simulink model "TRN_V3_CodeGen"  (R2022a)
settings: Solver=FixedStepAuto  StartTime=0.0  StopTime=300  FixedStep=0.04  RelTol=1e-3
PreLoadFcn:
  | % Add DataBus Path
  | addpath(',/TRN');
  | addpath('./MAP/');
  | addpath('./MAP/MAP_DB');
  | addpath('./MAP/DVOF');
  | addpath(genpath(cd));
  | load('BusStructureTRN.mat');
InitFcn:
  | % Add DataBus Path
  | addpath(',/TRN');
  | addpath('./MAP/');
  | addpath('./MAP/MAP_DB');
  | addpath('./MAP/DVOF');
  | addpath(genpath(cd));
  | load('BusStructureTRN.mat');
undefined symbols (not defined in the file or in its folder): Altitude_INS, INSDataNotValid, Latitude_INS, Longitude_INS, RALTValid, TRN, TRNlib
libraries: simulink_extras x33, aerolibconvert2 x6, dspstat3 x3, sharedtransform x2
(part 2 of 3)

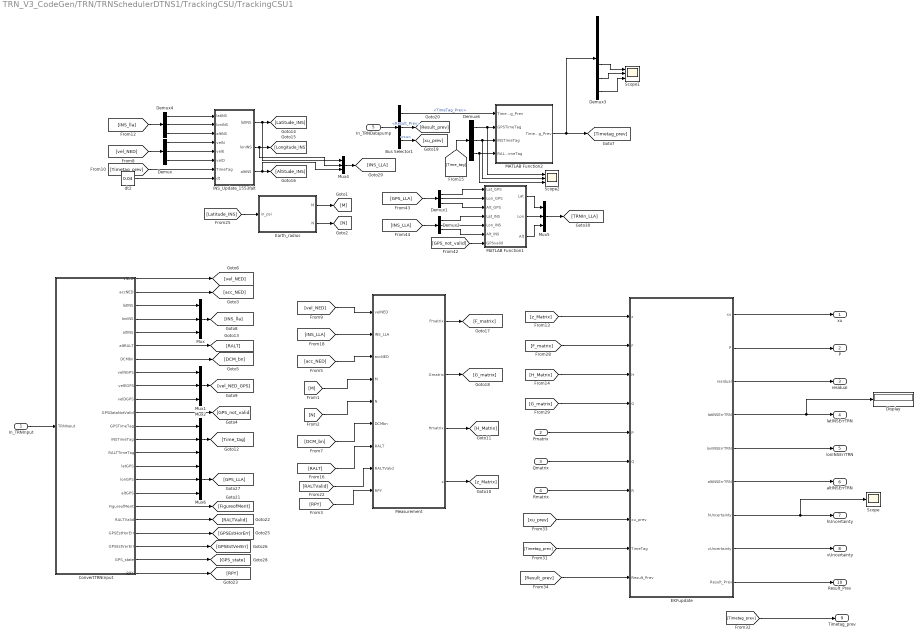
== system TRN_V3_CodeGen/TRN/TRNSchedulerDTNS1/TrackingCSU/TrackingCSU1 ==
  In_TRNInput : Inport  OutDataTypeStr=Bus: TRNInput
  Pmatrix : Inport  Port=2
  Qmatrix : Inport  Port=3
  Rmatrix : Inport  Port=4
  In_TRNDatapump : Inport  Port=5  OutDataTypeStr=Bus: TRNDatapump  PortDimensions=1
  Bus Selector1 : BusSelector  OutputSignals=TimeTag_Prev,Result_Prev,xu
  ConvertTRNInput : Subsystem  TreatAsAtomicUnit=on
  Demux{,1..2,4,6} (5 alike) : Demux  Outputs=3
  Demux3 : Demux  Outputs=6
  Display : Display
  EKFupdate : Subsystem
  Earth_radius : MATLAB Function  TreatAsAtomicUnit=on
  INS_Update_1553falt : MATLAB Function  TreatAsAtomicUnit=on
  MATLAB Function1 : MATLAB Function  TreatAsAtomicUnit=on
  MATLAB Function2 : MATLAB Function  TreatAsAtomicUnit=on
  Measurement : Subsystem
  Mux{,1..2,4..6} (6 alike) : Mux  Inputs=3
  Scope : Scope
  Scope1 : Scope  NumInputPorts=3
  Scope2 : Scope  NumInputPorts=3
  dt2 : Constant  Value=0.04  OutDataTypeStr=double
  xu : Outport
  P : Outport  Port=2
  residual : Outport  Port=3
  latINSErrTRN : Outport  Port=4
  lonINSErrTRN : Outport  Port=5
  altINSErrTRN : Outport  Port=6
  hUncertainty : Outport  Port=7
  vUncertainty : Outport  Port=8
  Timetag_prev : Outport  Port=9
  Result_Prev : Outport  Port=10
  wires:
  Mux5/1 -> [TRNIn_LLA]
  MATLAB Function1/3(Alt) -> Mux5/3
  MATLAB Function1/1(Lat) -> Mux5/1
  MATLAB Function1/2(Lon) -> Mux5/2
  Demux2/3 -> MATLAB Function1/6(Alt_INS)
  Demux2/2 -> MATLAB Function1/5(Lon_INS)
  Demux2/1 -> MATLAB Function1/4(Lat_INS)
  [INS_LLA] -> Demux2/1
  Mux4/1 -> [INS_LLA]
  Demux1/3 -> MATLAB Function1/3(Alt_GPS)
  Demux1/1 -> MATLAB Function1/1(Lat_GPS)
  Demux1/2 -> MATLAB Function1/2(Lon_GPS)
  [GPS_LLA] -> Demux1/1
  [GPS_not_valid] -> MATLAB Function1/7(GPSvalid)
  ConvertTRNInput/22(GPS_state) -> [GPS_state]
  ConvertTRNInput/21(GPSEstVerErr) -> [GPSEstVerErr]
  ConvertTRNInput/20(GPSEstHorErr) -> [GPSEstHorErr]
  Demux/3 -> INS_Update_1553falt/6(velD)
  Demux/1 -> INS_Update_1553falt/4(velN)
  Demux/2 -> INS_Update_1553falt/5(velE)
  dt2/1 -> INS_Update_1553falt/8(dt)
  Bus Selector1/1 -> MATLAB Function2/1("TimeTag_Prev ")  "<TimeTag_Prev>"
  In_TRNDatapump/1 -> Bus Selector1/1
  INS_Update_1553falt/3(altINS) -> [Altitude_INS], Mux4/3
  In_TRNInput/1 -> ConvertTRNInput/1(TRNInput)
  INS_Update_1553falt/1(latINS) -> [Latitude_INS], Mux4/1
  INS_Update_1553falt/2(lonINS) -> [Longitude_INS], Mux4/2
  ConvertTRNInput/2(accNED) -> [acc_NED]
  ConvertTRNInput/11(GPSDataNotValid) -> [GPS_not_valid]
  ConvertTRNInput/7(DCMbn) -> [DCM_bn]
  ConvertTRNInput/1(vNED) -> [vel_NED]
  [vel_NED] -> Demux/1
  [Timetag_prev] -> INS_Update_1553falt/7(TimeTag)
  ConvertTRNInput/3(latINS) -> Mux/1
  ConvertTRNInput/4(lonINS) -> Mux/2
  ConvertTRNInput/5(altINS) -> Mux/3
  Mux/1 -> [INS_lla]
  [INS_lla] -> Demux4/1
  Demux4/2 -> INS_Update_1553falt/2("lonINS ")
  Demux4/1 -> INS_Update_1553falt/1("latINS ")
  Demux4/3 -> INS_Update_1553falt/3("altINS ")
  ConvertTRNInput/10(velDGPS) -> Mux1/3
  ConvertTRNInput/9(velEGPS) -> Mux1/2
  Mux1/1 -> [vel_NED_GPS]
  ConvertTRNInput/8(velNGPS) -> Mux1/1
  Mux2/1 -> [Time_tag]
  ConvertTRNInput/12(GPSTimeTag) -> Mux2/1
  ConvertTRNInput/13(INSTimeTag) -> Mux2/2
  ConvertTRNInput/14(RALTTimeTag) -> Mux2/3
  [Time_tag] -> Demux6/1
  Demux6/1 -> Scope2/1, MATLAB Function2/2(GPSTimeTag)
  Demux6/2 -> Scope2/2, MATLAB Function2/3(INSTimeTag)
  Demux6/3 -> Scope2/3, MATLAB Function2/4(RALTTimeTag)
  ConvertTRNInput/6(altRALT) -> [RALT]
  [Timetag_prev] -> Timetag_prev/1
  Bus Selector1/3 -> [xu_prev]  "<xu>"
  Bus Selector1/2 -> [Result_prev]  "<Result_Prev>"
  Measurement/1(Fmatrix) -> [F_matrix]
  Measurement/2(Gmatrix) -> [G_matrix]
  Measurement/3(Hmatrix) -> [H_Matrix]
  Measurement/4(z) -> [z_Matrix]
  [z_Matrix] -> EKFupdate/1(z)
  [F_matrix] -> EKFupdate/2(F)
  [H_Matrix] -> EKFupdate/3(H)
  [G_matrix] -> EKFupdate/4(G)
  Pmatrix/1 -> EKFupdate/5("P ")
  Qmatrix/1 -> EKFupdate/6(Q)
  Rmatrix/1 -> EKFupdate/7(R)
  [xu_prev] -> EKFupdate/8(xu_prev)
  [Timetag_prev] -> EKFupdate/9(TimeTag)
  [Result_prev] -> EKFupdate/10("Result_Prev ")
  EKFupdate/1(xu) -> xu/1
  EKFupdate/2(P) -> P/1
  EKFupdate/3(residual) -> residual/1
  EKFupdate/8(vUncertainty) -> vUncertainty/1
  EKFupdate/4(latINSErrTRN) -> Display/1, latINSErrTRN/1
  EKFupdate/5(lonINSErrTRN) -> lonINSErrTRN/1
  EKFupdate/6(altINSErrTRN) -> altINSErrTRN/1
  EKFupdate/9(Result_Prev) -> Result_Prev/1
  ConvertTRNInput/18(FigureofMerit) -> [FigureofMerit]
  EKFupdate/7(hUncertainty) -> Scope/1, hUncertainty/1
  ConvertTRNInput/19(RALTValid) -> [RALTValid]
  [RALTValid] -> Measurement/8(RALTValid)
  [vel_NED] -> Measurement/1(velNED)
  [INS_LLA] -> Measurement/2(INS_LLA)
  [acc_NED] -> Measurement/3(accNED)
  [M] -> Measurement/4(M)
  [N] -> Measurement/5(N)
  [Latitude_INS] -> Earth_radius/1(in_psi)
  Earth_radius/1(M) -> [M]
  Earth_radius/2(N) -> [N]
  ConvertTRNInput/15(latGPS) -> Mux6/1
  ConvertTRNInput/16(lonGPS) -> Mux6/2
  ConvertTRNInput/17(altGPS) -> Mux6/3
  Mux6/1 -> [GPS_LLA]
  [RALT] -> Measurement/7(RALT)
  [DCM_bn] -> Measurement/6(DCMbn)
  ConvertTRNInput/23(RPY) -> [RPY]
  [RPY] -> Measurement/9(RPY)
  MATLAB Function2/1(TimeTag_Prev) -> Demux3/1, [Timetag_prev]
  Demux3/4 -> Scope1/1
  Demux3/5 -> Scope1/2
  Demux3/6 -> Scope1/3

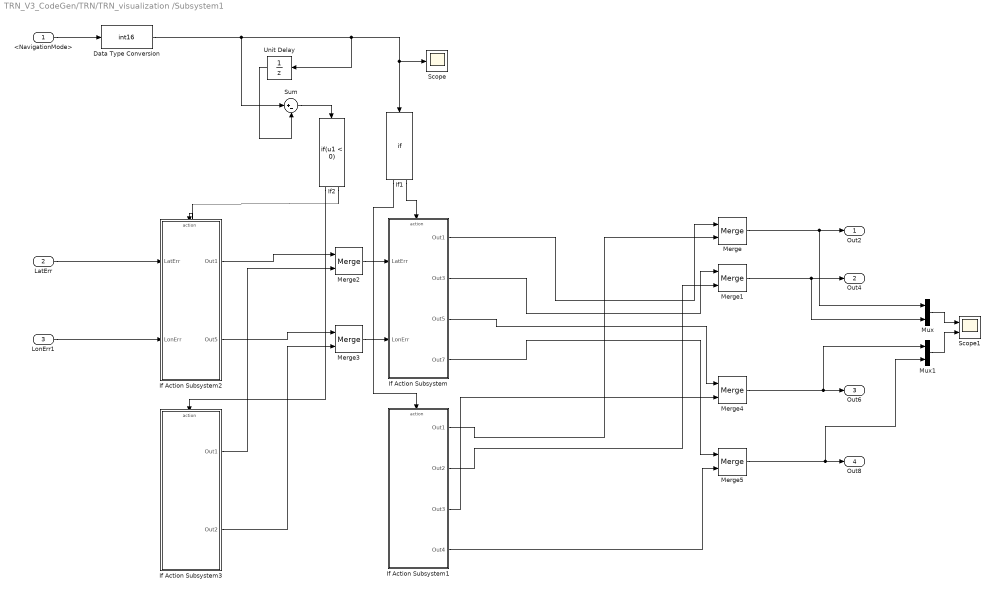
== system TRN_V3_CodeGen/TRN/TRN_visualization /Subsystem1 ==
  <NavigationMode> : Inport
  LatErr : Inport  Port=2
  LonErr1 : Inport  Port=3
  Data Type Conversion : DataTypeConversion  OutDataTypeStr=int16  SaturateOnIntegerOverflow=off  RndMeth=Floor
  If Action Subsystem : Subsystem  TreatAsAtomicUnit=on
  If Action Subsystem1 : Subsystem  TreatAsAtomicUnit=on
  If Action Subsystem2 : Subsystem  TreatAsAtomicUnit=on
  If Action Subsystem3 : Subsystem  TreatAsAtomicUnit=on
  If1 : If
  If2 : If  IfExpression=u1 < 0
  Merge{,1..5} (6 alike) : Merge
  Mux : Mux  Inputs=2
  Mux1 : Mux  Inputs=2
  Scope : Scope
  Scope1 : Scope  NumInputPorts=2
  Sum : Sum  Inputs=|+-
  Unit Delay : UnitDelay  SampleTime=-1  HasFrameUpgradeWarning=on
  Out2 : Outport
  Out4 : Outport  Port=2
  Out6 : Outport  Port=3
  Out8 : Outport  Port=4
  wires:
  If Action Subsystem3/2(Out2) -> Merge3/2
  If Action Subsystem2/2(Out5) -> Merge3/1
  If Action Subsystem3/1(Out1) -> Merge2/2
  If Action Subsystem2/1(Out1) -> Merge2/1
  Merge3/1 -> If Action Subsystem/2(LonErr)
  Merge2/1 -> If Action Subsystem/1(LatErr)
  LonErr1/1 -> If Action Subsystem2/2(LonErr)
  LatErr/1 -> If Action Subsystem2/1(LatErr)
  If2/1 -> If Action Subsystem3/Action
  If2/2 -> If Action Subsystem2/Action
  Sum/1 -> If2/1
  Unit Delay/1 -> Sum/2
  Mux1/1 -> Scope1/2
  Mux/1 -> Scope1/1
  <NavigationMode>/1 -> Data Type Conversion/1
  If Action Subsystem1/4(Out4) -> Merge5/2
  If Action Subsystem1/3(Out3) -> Merge4/2
  If Action Subsystem/4(Out7) -> Merge5/1
  If Action Subsystem/3(Out5) -> Merge4/1
  If Action Subsystem/2(Out3) -> Merge1/1
  Merge1/1 -> Out4/1, Mux/2
  Merge/1 -> Out2/1, Mux/1
  If1/1 -> If Action Subsystem1/Action
  If Action Subsystem1/1(Out1) -> Merge/2
  If Action Subsystem1/2(Out2) -> Merge1/2
  Data Type Conversion/1 -> Sum/1, Scope/1, If1/1, Unit Delay/1
  Merge4/1 -> Out6/1, Mux1/1
  Merge5/1 -> Out8/1, Mux1/2
  If1/2 -> If Action Subsystem/Action
  If Action Subsystem/1(Out1) -> Merge/1

== system TRN_V3_CodeGen/TRN/TRNSchedulerDTNS1/AcquisitionCSU/AcquisitionCSU/ConvertTRNInput ==
  TRNInput : Inport  OutDataTypeStr=Bus: TRNInput
  Bus Selector1 : BusSelector  OutputSignals=Latitude_INS,Longitude_INS,Altitude_INS,RALTAltitude,GPSDataNotValid,Latitude_GPS,Longitude_GPS,Altitude_GPS,INSDataNotValid
  Degrees to Radians{1..2,4..5} (4 alike) : simulink_extras/Transformations/Degrees to Radians
  latINS : Outport  VectorParamsAs1DForOutWhenUnconnected=off
  lonINS : Outport  Port=2  VectorParamsAs1DForOutWhenUnconnected=off
  altINS : Outport  Port=3  VectorParamsAs1DForOutWhenUnconnected=off
  altRALT : Outport  Port=4  VectorParamsAs1DForOutWhenUnconnected=off
  latGPS : Outport  Port=5  VectorParamsAs1DForOutWhenUnconnected=off
  lonGPS : Outport  Port=6  VectorParamsAs1DForOutWhenUnconnected=off
  altGPS : Outport  Port=7  VectorParamsAs1DForOutWhenUnconnected=off
  flagGPS : Outport  Port=8  VectorParamsAs1DForOutWhenUnconnected=off
  flagINS : Outport  Port=9  VectorParamsAs1DForOutWhenUnconnected=off
  wires:
  Bus Selector1/9 -> flagINS/1  "<INSDataNotValid>"
  Bus Selector1/2 -> Degrees to Radians4/1  "<Longitude_INS>"
  Bus Selector1/1 -> Degrees to Radians5/1  "<Latitude_INS>"
  Bus Selector1/4 -> altRALT/1  "<RALTAltitude>"
  Degrees to Radians4/1 -> lonINS/1
  Degrees to Radians5/1 -> latINS/1
  TRNInput/1 -> Bus Selector1/1
  Bus Selector1/3 -> altINS/1  "<Altitude_INS>"
  Bus Selector1/5 -> flagGPS/1  "<GPSDataNotValid>"
  Bus Selector1/6 -> Degrees to Radians1/1  "<Latitude_GPS>"
  Bus Selector1/7 -> Degrees to Radians2/1  "<Longitude_GPS>"
  Bus Selector1/8 -> altGPS/1  "<Altitude_GPS>"
  Degrees to Radians2/1 -> lonGPS/1
  Degrees to Radians1/1 -> latGPS/1

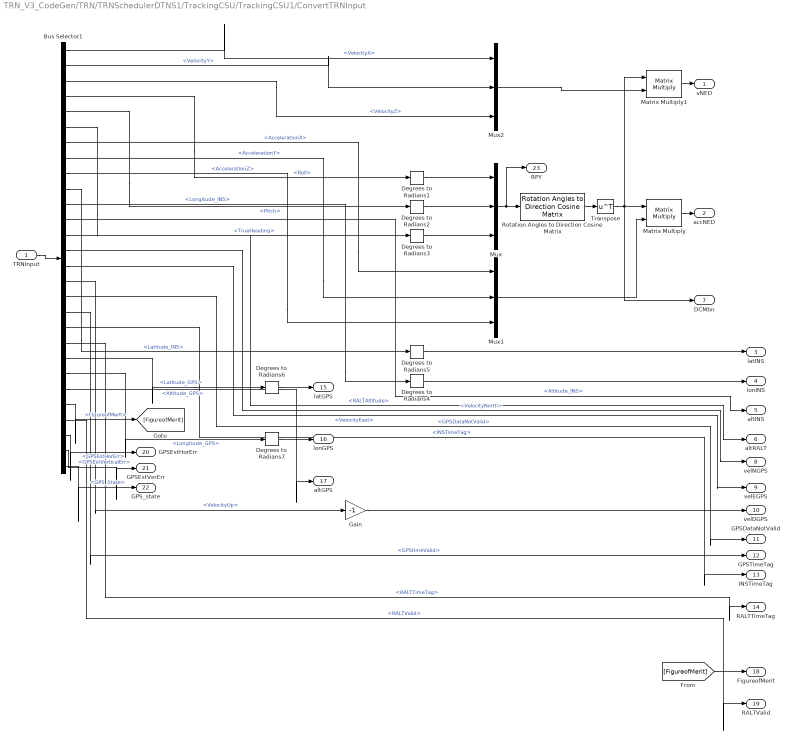
== system TRN_V3_CodeGen/TRN/TRNSchedulerDTNS1/TrackingCSU/TrackingCSU1/ConvertTRNInput ==
  TRNInput : Inport
  Bus Selector1 : BusSelector  OutputSignals=VelocityX,VelocityY,VelocityZ,Roll,Pitch,TrueHeading,AccelerationX,AccelerationY,AccelerationZ,Latitude_INS,Longitude_INS,Altitude_INS,RALTAltitude,VelocityNorth,VelocityEast,VelocityUp,GPSDataNotValid,GPStimeValid,INSTimeTag,RALTTimeTag,Latitude_GPS,Longitude_GPS,Altitude_GPS,FigureofMerit,RALTValid,GPSEstHorErr,GPSEstVerticalErr,GPS_State
  Degrees to Radians{1..7} (7 alike) : simulink_extras/Transformations/Degrees to Radians
  Gain : Gain  Gain=-1
  Matrix Multiply : Product  Multiplication=Matrix(*)
  Matrix Multiply1 : Product  Multiplication=Matrix(*)
  Mux : Mux  Inputs=3
  Mux1 : Mux  Inputs=3
  Mux2 : Mux  Inputs=3
  Rotation Angles to Direction Cosine Matrix : sharedtransform/Rotation Angles to Direction Cosine Matrix  rotationOrder=ZYX  aMode=aMode
      settings: SourceProductBaseCode=AE,PW,DR,MT,VE
  Transpose : Math  Operator=transpose  SignedPower=on
  vNED : Outport  VectorParamsAs1DForOutWhenUnconnected=off
  accNED : Outport  Port=2  VectorParamsAs1DForOutWhenUnconnected=off
  latINS : Outport  Port=3  VectorParamsAs1DForOutWhenUnconnected=off
  lonINS : Outport  Port=4  VectorParamsAs1DForOutWhenUnconnected=off
  altINS : Outport  Port=5  VectorParamsAs1DForOutWhenUnconnected=off
  altRALT : Outport  Port=6  VectorParamsAs1DForOutWhenUnconnected=off
  DCMbn : Outport  Port=7  VectorParamsAs1DForOutWhenUnconnected=off
  velNGPS : Outport  Port=8  VectorParamsAs1DForOutWhenUnconnected=off
  velEGPS : Outport  Port=9  VectorParamsAs1DForOutWhenUnconnected=off
  velDGPS : Outport  Port=10  VectorParamsAs1DForOutWhenUnconnected=off
  GPSDataNotValid : Outport  Port=11  VectorParamsAs1DForOutWhenUnconnected=off
  GPSTimeTag : Outport  Port=12  VectorParamsAs1DForOutWhenUnconnected=off
  INSTimeTag : Outport  Port=13  VectorParamsAs1DForOutWhenUnconnected=off
  RALTTimeTag : Outport  Port=14  VectorParamsAs1DForOutWhenUnconnected=off
  latGPS : Outport  Port=15
  lonGPS : Outport  Port=16
  altGPS : Outport  Port=17
  FigureofMerit : Outport  Port=18
  RALTValid : Outport  Port=19
  GPSEstHorErr : Outport  Port=20
  GPSEstVerErr : Outport  Port=21
  GPS_state : Outport  Port=22
  RPY : Outport  Port=23  VectorParamsAs1DForOutWhenUnconnected=off
  wires:
  Bus Selector1/28 -> GPS_state/1  "<GPS_State>"
  Bus Selector1/27 -> GPSEstVerErr/1  "<GPSEstVerticalErr>"
  Bus Selector1/26 -> GPSEstHorErr/1  "<GPSEstHorErr>"
  Bus Selector1/23 -> altGPS/1  "<Altitude_GPS>"
  Bus Selector1/22 -> Degrees to Radians7/1  "<Longitude_GPS>"
  Degrees to Radians7/1 -> lonGPS/1
  Bus Selector1/20 -> RALTTimeTag/1  "<RALTTimeTag>"
  Bus Selector1/19 -> INSTimeTag/1  "<INSTimeTag>"
  Bus Selector1/18 -> GPSTimeTag/1  "<GPStimeValid>"
  Bus Selector1/17 -> GPSDataNotValid/1  "<GPSDataNotValid>"
  Gain/1 -> velDGPS/1
  Bus Selector1/16 -> Gain/1  "<VelocityUp>"
  Bus Selector1/15 -> velEGPS/1  "<VelocityEast>"
  Bus Selector1/14 -> velNGPS/1  "<VelocityNorth>"
  Bus Selector1/12 -> altINS/1  "<Altitude_INS>"
  Bus Selector1/3 -> Mux2/3  "<VelocityZ>"
  Bus Selector1/1 -> Mux2/1  "<VelocityX>"
  Bus Selector1/4 -> Degrees to Radians1/1  "<Roll>"
  Bus Selector1/2 -> Mux2/2  "<VelocityY>"
  TRNInput/1 -> Bus Selector1/1
  Bus Selector1/6 -> Degrees to Radians3/1  "<TrueHeading>"
  Degrees to Radians2/1 -> Mux/2
  Degrees to Radians3/1 -> Mux/3
  Mux/1 -> RPY/1, Rotation Angles to Direction Cosine Matrix/1
  Bus Selector1/7 -> Mux1/1  "<AccelerationX>"
  Bus Selector1/5 -> Degrees to Radians2/1  "<Pitch>"
  Degrees to Radians1/1 -> Mux/1
  Bus Selector1/9 -> Mux1/3  "<AccelerationZ>"
  Bus Selector1/8 -> Mux1/2  "<AccelerationY>"
  Degrees to Radians5/1 -> latINS/1
  Matrix Multiply1/1 -> vNED/1
  Degrees to Radians4/1 -> lonINS/1
  Matrix Multiply/1 -> accNED/1
  Bus Selector1/13 -> altRALT/1  "<RALTAltitude>"
  Mux1/1 -> Matrix Multiply/2
  Bus Selector1/10 -> Degrees to Radians5/1  "<Latitude_INS>"
  Transpose/1 -> Matrix Multiply1/1, Matrix Multiply/1, DCMbn/1
  Mux2/1 -> Matrix Multiply1/2
  Rotation Angles to Direction Cosine Matrix/1 -> Transpose/1
  Bus Selector1/11 -> Degrees to Radians4/1  "<Longitude_INS>"
  Degrees to Radians6/1 -> latGPS/1
  Bus Selector1/21 -> Degrees to Radians6/1  "<Latitude_GPS>"
  Bus Selector1/24 -> [FigureofMerit]  "<FigureofMerit>"
  [FigureofMerit] -> FigureofMerit/1
  Bus Selector1/25 -> RALTValid/1  "<RALTValid>"

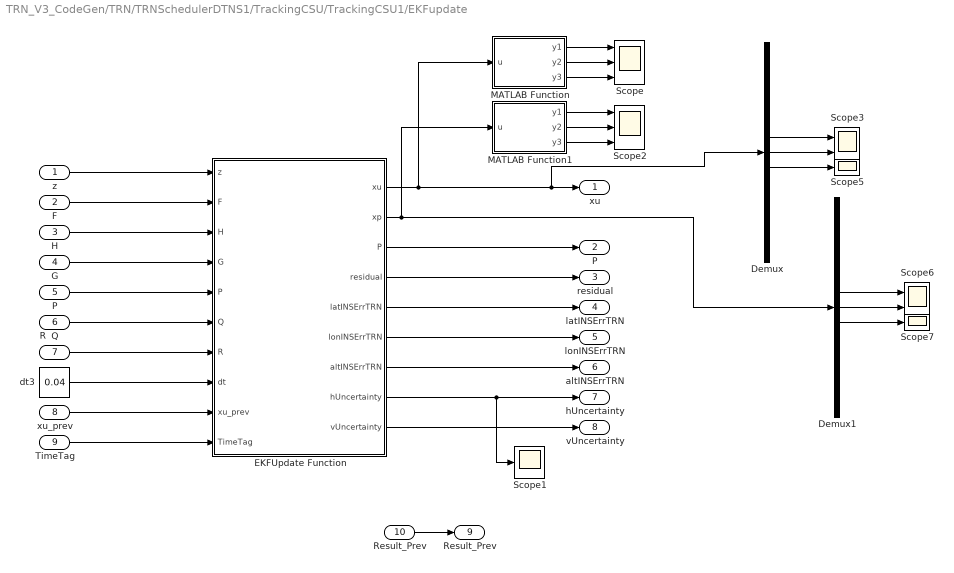
== system TRN_V3_CodeGen/TRN/TRNSchedulerDTNS1/TrackingCSU/TrackingCSU1/EKFupdate ==
  z : Inport
  F : Inport  Port=2
  H : Inport  Port=3
  G : Inport  Port=4
  "P " : Inport  Port=5
  Q : Inport  Port=6
  R : Inport  Port=7
  xu_prev : Inport  Port=8
  TimeTag : Inport  Port=9
  "Result_Prev " : Inport  Port=10
  Demux : Demux  Outputs=15
  Demux1 : Demux  Outputs=15
  EKFUpdate Function : MATLAB Function  TreatAsAtomicUnit=on
  MATLAB Function : MATLAB Function  TreatAsAtomicUnit=on
  MATLAB Function1 : MATLAB Function  TreatAsAtomicUnit=on
  Scope : Scope  NumInputPorts=3
  Scope1 : Scope
  Scope2 : Scope  NumInputPorts=3
  Scope3 : Scope  NumInputPorts=2
  Scope5 : Scope
  Scope6 : Scope  NumInputPorts=2
  Scope7 : Scope
  dt3 : Constant  Value=0.04  OutDataTypeStr=double
  xu : Outport
  P : Outport  Port=2
  residual : Outport  Port=3
  latINSErrTRN : Outport  Port=4
  lonINSErrTRN : Outport  Port=5
  altINSErrTRN : Outport  Port=6
  hUncertainty : Outport  Port=7
  vUncertainty : Outport  Port=8
  Result_Prev : Outport  Port=9
  wires:
  R/1 -> EKFUpdate Function/7(R)
  H/1 -> EKFUpdate Function/3(H)
  "P "/1 -> EKFUpdate Function/5("P ")
  EKFUpdate Function/9(vUncertainty) -> vUncertainty/1
  EKFUpdate Function/4(residual) -> residual/1
  TimeTag/1 -> EKFUpdate Function/10(TimeTag)
  F/1 -> EKFUpdate Function/2(F)
  xu_prev/1 -> EKFUpdate Function/9(xu_prev)
  G/1 -> EKFUpdate Function/4(G)
  EKFUpdate Function/1(xu) -> MATLAB Function/1(u), Demux/1, xu/1
  EKFUpdate Function/3(P) -> P/1
  Q/1 -> EKFUpdate Function/6(Q)
  z/1 -> EKFUpdate Function/1(z)
  dt3/1 -> EKFUpdate Function/8(dt)
  EKFUpdate Function/5(latINSErrTRN) -> latINSErrTRN/1
  EKFUpdate Function/6(lonINSErrTRN) -> lonINSErrTRN/1
  EKFUpdate Function/7(altINSErrTRN) -> altINSErrTRN/1
  EKFUpdate Function/8(hUncertainty) -> Scope1/1, hUncertainty/1
  "Result_Prev "/1 -> Result_Prev/1
  MATLAB Function/1(y1) -> Scope/1
  MATLAB Function/2(y2) -> Scope/2
  MATLAB Function/3(y3) -> Scope/3
  MATLAB Function1/1(y1) -> Scope2/1
  MATLAB Function1/2(y2) -> Scope2/2
  MATLAB Function1/3(y3) -> Scope2/3
  Demux/7 -> Scope3/1
  Demux/8 -> Scope3/2
  EKFUpdate Function/2(xp) -> MATLAB Function1/1(u), Demux1/1
  Demux/9 -> Scope5/1
  Demux1/9 -> Scope7/1
  Demux1/8 -> Scope6/2
  Demux1/7 -> Scope6/1

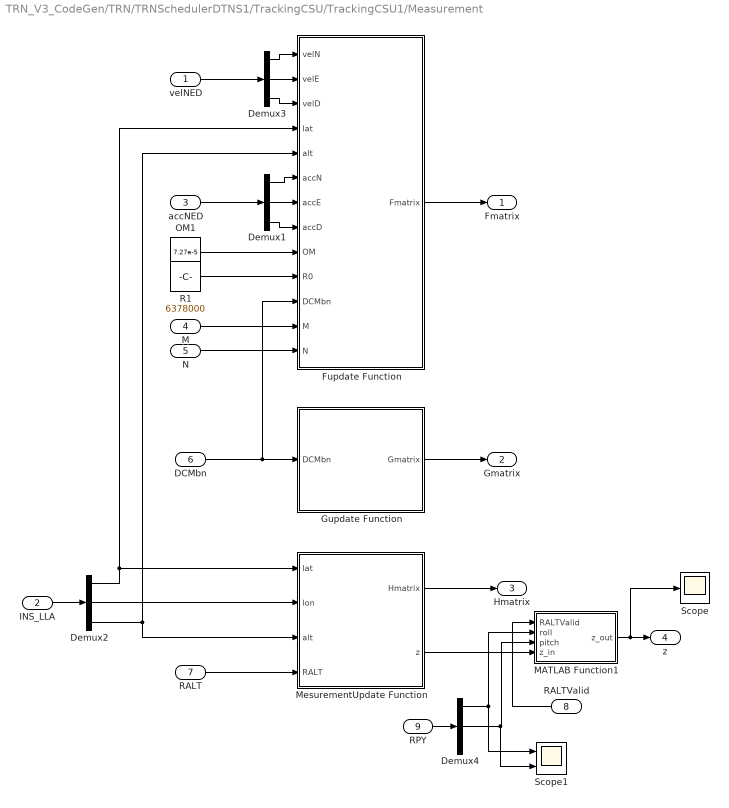
== system TRN_V3_CodeGen/TRN/TRNSchedulerDTNS1/TrackingCSU/TrackingCSU1/Measurement ==
  velNED : Inport
  INS_LLA : Inport  Port=2
  accNED : Inport  Port=3
  M : Inport  Port=4
  N : Inport  Port=5
  DCMbn : Inport  Port=6
  RALT : Inport  Port=7
  RALTValid : Inport  Port=8
  RPY : Inport  Port=9
  Demux{1..4} (4 alike) : Demux  Outputs=3
  Fupdate Function : MATLAB Function  TreatAsAtomicUnit=on
  Gupdate Function : MATLAB Function  TreatAsAtomicUnit=on
  MATLAB Function1 : MATLAB Function  TreatAsAtomicUnit=on
  MesurementUpdate Function : MATLAB Function  TreatAsAtomicUnit=on
  OM1 : Constant  Value=7.27e-5
  R1 : Constant  Value=6378000
  Scope : Scope
  Scope1 : Scope  NumInputPorts=2
  Fmatrix : Outport
  Gmatrix : Outport  Port=2
  Hmatrix : Outport  Port=3
  z : Outport  Port=4
  wires:
  Demux1/3 -> Fupdate Function/8(accD)
  OM1/1 -> Fupdate Function/9(OM)
  Demux3/1 -> Fupdate Function/1(velN)
  Demux1/2 -> Fupdate Function/7(accE)
  RALT/1 -> MesurementUpdate Function/4(RALT)
  Demux3/3 -> Fupdate Function/3(velD)
  Demux3/2 -> Fupdate Function/2(velE)
  Demux1/1 -> Fupdate Function/6(accN)
  Gupdate Function/1(Gmatrix) -> Gmatrix/1
  Fupdate Function/1(Fmatrix) -> Fmatrix/1
  DCMbn/1 -> Fupdate Function/11(DCMbn), Gupdate Function/1(DCMbn)
  N/1 -> Fupdate Function/13(N)
  accNED/1 -> Demux1/1
  velNED/1 -> Demux3/1
  M/1 -> Fupdate Function/12(M)
  MesurementUpdate Function/1(Hmatrix) -> Hmatrix/1
  R1/1 -> Fupdate Function/10(R0)
  RALTValid/1 -> MATLAB Function1/1(RALTValid)
  MesurementUpdate Function/2(z) -> MATLAB Function1/4(z_in)
  INS_LLA/1 -> Demux2/1
  Demux2/1 -> Fupdate Function/4(lat), MesurementUpdate Function/1(lat)
  Demux2/3 -> MesurementUpdate Function/3(alt), Fupdate Function/5(alt)
  Demux2/2 -> MesurementUpdate Function/2(lon)
  RPY/1 -> Demux4/1
  Demux4/1 -> MATLAB Function1/2(roll), Scope1/1
  Demux4/2 -> Scope1/2, MATLAB Function1/3(pitch)
  MATLAB Function1/1(z_out) -> z/1, Scope/1

== system TRN_V3_CodeGen/TRN/TRN_visualization /Subsystem1/If Action Subsystem ==
  LatErr : Inport
  LonErr : Inport  Port=2
  Action Port : ActionPort  ActionPortLabel=else
  Gain1 : Gain  Gain=3
  Gain2 : Gain  Gain=3
  Gain3 : Gain
  Gain4 : Gain  Gain=-1
  Gain6 : Gain
  Gain7 : Gain  Gain=-1
  Standard Deviation : dspstat3/Standard Deviation  run=on  directionMode=Entire input  dimension=1  reset_popup=None  roiEnable=off  roiType=Rectangles  roiPortion=Entire ROI  roiOutput=Individual statistics for each ROI  roiFlag=off
      settings: SourceProductBaseCode=DS
  Standard Deviation1 : dspstat3/Standard Deviation  run=on  directionMode=Entire input  dimension=1  reset_popup=None  roiEnable=off  roiType=Rectangles  roiPortion=Entire ROI  roiOutput=Individual statistics for each ROI  roiFlag=off
      settings: SourceProductBaseCode=DS
  Out1 : Outport
  Out3 : Outport  Port=2
  Out5 : Outport  Port=3
  Out7 : Outport  Port=4
  wires:
  LatErr/1 -> Standard Deviation/1
  LonErr/1 -> Standard Deviation1/1
  Gain6/1 -> Out5/1
  Gain2/1 -> Gain4/1, Gain3/1
  Gain7/1 -> Out7/1
  Standard Deviation1/1 -> Gain1/1
  Standard Deviation/1 -> Gain2/1
  Gain3/1 -> Out1/1
  Gain4/1 -> Out3/1
  Gain1/1 -> Gain7/1, Gain6/1

== system TRN_V3_CodeGen/TRN/TRN_visualization /Subsystem1/If Action Subsystem1 ==
  Action Port : ActionPort  ActionPortLabel=if(u1 > 0)
  Constant : Constant  Value=0
  Out1 : Outport
  Out2 : Outport  Port=2
  Out3 : Outport  Port=3
  Out4 : Outport  Port=4
  wires:
  Constant/1 -> Out4/1, Out3/1, Out2/1, Out1/1

== system TRN_V3_CodeGen/TRN/TRN_visualization /Subsystem1/If Action Subsystem2 ==
  LatErr : Inport
  LonErr : Inport  Port=2
  Action Port : ActionPort  ActionPortLabel=else
  Out1 : Outport
  Out5 : Outport  Port=2
  wires:
  LonErr/1 -> Out5/1
  LatErr/1 -> Out1/1

== system TRN_V3_CodeGen/TRN/TRN_visualization /Subsystem1/If Action Subsystem3 ==
  Action Port : ActionPort  ActionPortLabel=if(u1 < 0)
  Constant : Constant  Value=0
  Out1 : Outport
  Out2 : Outport  Port=2
  wires:
  Constant/1 -> Out2/1, Out1/1

== matlab function TRN_V3_CodeGen/TRN/INS//GPSFilter/MATLAB Function2 ==
  data: FoM input; out_GPSpos output; EstHorErr input; EstVerErr input; state input; in_GPSpos input; in_GPSvel input; out_GPSvel output; GPSDataNotValid input
function [out_GPSpos, out_GPSvel] = GPScheck(FoM, EstHorErr, EstVerErr, state, in_GPSpos, in_GPSvel, GPSDataNotValid)

if GPSDataNotValid == 0
    if EstHorErr < 100 && EstVerErr < 25 && state == 5
        if FoM < 4
            out_GPSpos = in_GPSpos;
            out_GPSvel = zeros(3,1);
            if FoM < 2
                out_GPSpos = in_GPSpos;
                out_GPSvel = in_GPSvel;
            end
        else
            out_GPSpos = zeros(3,1);
            out_GPSvel = zeros(3,1);
        end
    else
        out_GPSpos = zeros(3,1);
        out_GPSvel = zeros(3,1);
    end
else
    out_GPSpos = zeros(3,1);
    out_GPSvel = zeros(3,1);
end

== matlab function TRN_V3_CodeGen/TRN/MATLAB Function ==
  data: u input; yy output
function yy = fcn(u)
    y = diag(u);
    yy = [y(7), y(8), y(9)./(6378000)];

    yy = yy.*(6378000*25);

end

== matlab function TRN_V3_CodeGen/TRN/MATLAB Function1 ==
  data: latINS input; TRNEstOfLatErr output; lonINS input; altINS input; latGPS input; lonGPS input; altGPS input; flagGPS input; TRNEstOfLonErr output; TRNEstOfaltErr output; roll input; pitch input
function [TRNEstOfLatErr, TRNEstOfLonErr, TRNEstOfaltErr] = fcn(latINS, lonINS, altINS,  latGPS, lonGPS, altGPS, flagGPS, roll, pitch)

if abs(roll) < 15 && abs(pitch) < 15
    TRNEstOfLatErr = latINS;
    TRNEstOfLonErr = lonINS;
    TRNEstOfaltErr = altINS;
    if flagGPS ==0
      TRNEstOfLatErr = latGPS;
      TRNEstOfLonErr = lonGPS;
      TRNEstOfaltErr = altGPS;
    end
else
    TRNEstOfLatErr = 0;
    TRNEstOfLonErr = 0;
    TRNEstOfaltErr = 0;
end

== matlab function TRN_V3_CodeGen/TRN/MATLAB Function2 ==
  data: INS_Mech_flag input; TRN_valid output; Latitude_INS input
function TRN_valid = fcn(INS_Mech_flag, Latitude_INS)

    if( abs(Latitude_INS) > 80.0)
        Latitude_INS_flag = 0;
    else
        Latitude_INS_flag = 1;
    end

    if( (INS_Mech_flag < 1) || (Latitude_INS_flag < 1))
        TRN_valid = boolean(false);
    else
        TRN_valid = boolean(true);
    end

end

== matlab function TRN_V3_CodeGen/TRN/INS//GPSFilter/EKFUpdate Function ==
  data: xu input; xu output; z input; P_out output; F input; H input; G input; P input; Q input; R input; dt input; LCI_lat output; LCI_lon output; LCI_alt output
% function [xu, P, residual, LCI_lat, LCI_lon, LCI_alt] = EKFUpdate(z, F, H, G, P, Q, R, dt, xu_prev, TimeTag)
function [xu, P_out, LCI_lat, LCI_lon, LCI_alt] = EKFUpdate(xu, z, F, H, G, P, Q, R, dt)

x = xu;
I = eye(max(size(F)));

A = I + (F*dt);
Qk = (A*G * Q * G'*A') .* dt;

%-------------------------------------%
% Predicts states & covariance matrix
%-------------------------------------%
xp = A * x;
Pp = (A * P * A') + Qk;

%---------------------%
% Updates Kalman gain
%---------------------%
K = (Pp * H')/(R + H * Pp * H');

%----------------%
% Updates states
%----------------%
xu = xp + K * (z - H*xp);
% residual = z;

%---------------------------%
% Updates covariance matrix
%---------------------------%
% P_out = (I - K*H) * Pp * (I - K*H)' + K*R*K';
P_out = (I - K*H)*Pp;


LCI_lat = xu(1);
LCI_lon = xu(2);
LCI_alt = xu(3);
    
% if TimeTag(6) == 1
%     xu = xu_prev;
%     latINSErrTRN = xu(7);
%     lonINSErrTRN = xu(8);
%     altINSErrTRN = xu(9);
% end

end

== matlab function TRN_V3_CodeGen/TRN/MATLAB Function4 ==
  data: P input; hUncertainty output; vUncertainty output
function [hUncertainty,vUncertainty] = fcn(P)

hUncertainty = sqrt(abs(P(7,7) + P(8,8))) * 6378000;
vUncertainty = sqrt(abs(P(9,9)));

== matlab function TRN_V3_CodeGen/TRN/INSValidCheck/MATLAB Function5 ==
  data: diff_Lat input; NotValid output; diff_Lon input; Valid input; in_count input; out_count output
function [NotValid,out_count] = INSValidCheck(diff_Lat,diff_Lon,Valid,in_count)
out_count = 0;
NotValid = boolean(false);
lat2m = 111000;
lon2m = 91170;

if Valid == 0                       % INS Notvalid [5sec]
    NotValid = boolean(false);      % Init Setting
    out_count = in_count + 1;
    if out_count > (5*25)
        NotValid = boolean(true);   % INS Notvalid
    end
elseif (abs(diff_Lat*lat2m) > 100 || abs(diff_Lon*lon2m) > 100)                  % INS Switch
    NotValid = boolean(true);
elseif Valid > 0 && (abs(diff_Lat*lat2m) <= 100 && abs(diff_Lon*lon2m) <= 100)   % INS valid
    NotValid = boolean(false);                                                   % INS valid
end

== matlab function TRN_V3_CodeGen/TRN/Subsystem/FTGMapCaching ==
  data: resultDTED output; resultDVOF output; lat input; lon input; hDEM output
function [resultDTED, resultDVOF, hDEM] = FTGMapCaching(lat, lon)

persistent latPrev lonPrev

if isempty(latPrev)
    latPrev = 0.0;
end
if isempty(lonPrev)
    lonPrev = 0.0;
end

resultDTED = uint32(1);
resultDVOF = int32(1);
hDEM = double(0.0);                                 %%20220419


if ( abs(lat - latPrev) > 0.01 ) || ( abs(lon - lonPrev) > 0.01)
    resultDVOF = coder.ceval('UpdateObstList', lat, lon);
    resultDTED = coder.ceval('UpdateMapCache', lat, lon);
    latPrev = lat;
    lonPrev = lon;
else
    
end

hDEM = coder.ceval('GetElevation', lat, lon);       %%20220419

== matlab function TRN_V3_CodeGen/TRN/Subsystem/MATLAB Function ==
  data: Resolution output; Map_Size output; bottomLat output; leftLon output
function [Resolution, Map_Size, bottomLat, leftLon] = ReturnBottomLeftLatLon

Resolution = double(0.0);
Map_Size = double(0.0);

leftLon = 0.0;
leftLon = coder.ceval('ReturnLeftLon');

bottomLat = 0.0;
bottomLat = coder.ceval('ReturnBottomLat');

end

== matlab function TRN_V3_CodeGen/TRN/TRN_visualization /MATLAB Function ==
  data: Err_Lat_INS output; Err_Lon_INS output; Err_Alt_INS output; lat_Ref input; lon_Ref input; alt_Ref input; lat_INS input; lon_INS input; alt_INS input; Lat_INS output; Lon_INS output; Alt_INS output; Lat_Ref output; Lon_Ref output; Alt_Ref output
function [Err_Lat_INS, Err_Lon_INS, Err_Alt_INS, Lat_INS, Lon_INS, Alt_INS, Lat_Ref, Lon_Ref, Alt_Ref] = fcn(lat_Ref, lon_Ref, alt_Ref, lat_INS, lon_INS, alt_INS)

%% parameters
lat2m = 111000;
lon2m = 91170;

%% 초기값 setting
% init_lat = 35.1;
% init_lon = 128.5;
% init_alt = 1000;

Lat_INS = lat_INS;               % INS Latitude
Lon_INS = lon_INS;               % INS Longitude
% Alt_INS = uint16(alt_INS);               % INS Altitude
Alt_INS = alt_INS;               % INS Altitude

Lat_Ref = lat_Ref;             % Ref Latitude
Lon_Ref = lon_Ref;             % Ref Longitude
% Alt_Ref = uint16(alt_Ref);             % Ref Altitude
Alt_Ref = alt_Ref;             % Ref Altitude

Err_Lat_INS = (Lat_Ref-Lat_INS)*lat2m;
Err_Lon_INS = (Lon_Ref-Lon_INS)*lon2m;
Err_Alt_INS = (Alt_Ref-Alt_INS);

end

== matlab function TRN_V3_CodeGen/TRN/TRN_visualization /MATLAB Function1 ==
  data: x input; a output; y input
function a = fcn(x,y)

a = sqrt(x^2+y^2);

== matlab function TRN_V3_CodeGen/TRN/TRN_visualization /MATLAB Function2 ==
  data: x input; a output; y input
function a = fcn(x,y)

a = sqrt(x^2+y^2);

== matlab function TRN_V3_CodeGen/TRN/TRN_visualization /Terrain_Level_big4 ==
  data: Lat input; Lon input; R output
function R = Terrain_level_big1(Lat, Lon)

    R = Terrain_level(Lat, Lon);

end

== stateflow chart TRN_V3_CodeGen/TRN/TRNSchedulerDTNS1 ==
  state Operation_In_Flight
    state Check_On_Terrain_Map [parallel]
      en, du:  Out_TRNOutput.AircraftOffTerrainMap = CheckOffTerrainMap(In_TRNInput.Latitude_INS, In_TRNInput.Longitude_INS);
      settings: executionOrder=1
    state Terrain_Referenced_Navigation [parallel]
      settings: executionOrder=2
      state On_Terrain_Map
        state AcquisitionCSU
          state Batch_On
            state CollectProfile [parallel]
              en, du: [Out_TRNDatapump.MAD, Out_TRNDatapump.profileCnt, posUpdate, Out_TRNDatapump.residual] =...
              AcquisitionCSU(In_TRNInput,In_TRNDatapump)
              settings: executionOrder=1
            state CorrelationAnalysis [parallel]
              settings: executionOrder=2
              state BatchUpdate_On
                en, du: Out_TRNOutput.TRNEstOfINSLatitudeErr = -posUpdate(1) * 180/pi;
                Out_TRNOutput.TRNEstOfINSLongitudeErr = -posUpdate(2) * 180/pi;
                Out_TRNDatapump.profileCnt = 0;
                Out_TRNOutput.NavigationMode = false;
                Out_TRNOutput.AircraftPositionCorrectionValid = true;
                Out_Pmatrix = InitPmatrix();
              state BatchUpdate_Off
                en, du: Out_TRNOutput.TRNEstOfINSLatitudeErr = 0.0;
                Out_TRNOutput.TRNEstOfINSLongitudeErr = 0.0;
                Out_TRNOutput.NavigationMode = true;
                Out_TRNOutput.AircraftPositionCorrectionValid = false;
                Out_Pmatrix = InitPmatrix();
              (default) -> (junction 198)
              (junction 198) -> BatchUpdate_On [order 1] : [(Out_TRNDatapump.MAD <= 50&&...
                  | Out_TRNDatapump.profileCnt >= 20) || ...
                  |  (In_TRNInput.GPSDataNotValid == 0 && ...
                  | Out_TRNDatapump.MAD <= 50&&...
                  | Out_TRNDatapump.profileCnt >= 5)]
              (junction 198) -> BatchUpdate_Off [order 2]
          state Batch_Idle
            entry: Out_TRNOutput.TRNEstOfINSLatitudeErr = 0.0;
            Out_TRNOutput.TRNEstOfINSLongitudeErr = 0.0;
            Out_TRNOutput.NavigationMode = true;
            Out_TRNOutput.AircraftPositionCorrectionValid = false;
          (default) -> Batch_On
          Batch_Idle -> Batch_On : after(24, tick)
          Batch_On -> Batch_Idle : after(1, tick)
        state TrackingCSU
          state ContinuousUpdate [parallel]
            en,du:  [xu,Pmatrix,residual,latINSErrTRN,lonINSErrTRN, ...
            altINSErrTRN,hUncertainty,vUncertainty, Out_TRNDatapump.TimeTag_Prev, Out_TRNDatapump.Result_Prev] = ...
            TrackingCSU(In_TRNInput,In_Pmatrix,Qmatrix,Rmatrix, In_TRNDatapump);
            [continuousValid, Out_TRNOutput.NavigationMode]...
            = CheckValidity( hUncertainty, In_TRNInput.INSDataNotValid);
            settings: executionOrder=1
          state ValidityCheck [parallel]
            settings: executionOrder=2
            state ContinuousValid
              en, du:
              Out_TRNOutput.TRNEstOfINSLatitudeErr = latINSErrTRN * 180/pi;
              Out_TRNOutput.TRNEstOfINSLongitudeErr = lonINSErrTRN * 180/pi;
              Out_TRNOutput.TRNEstOfINSAltitudeErr = altINSErrTRN;
              Out_TRNOutput.AircraftPositionCorrectionValid = true;
            state ContinuousInValid
              en, du:
              Out_TRNOutput.TRNEstOfINSLatitudeErr = 0.0;
              Out_TRNOutput.TRNEstOfINSLongitudeErr = 0.0;
              Out_TRNOutput.TRNEstOfINSAltitudeErr = 0.0;
              Out_TRNOutput.AircraftPositionCorrectionValid = false;
            (default) -> ContinuousValid
            ContinuousValid -> ContinuousInValid : [continuousValid == false]
            ContinuousInValid -> ContinuousValid : [continuousValid == true]
          state UpdateContinuousParam [parallel]
            en, du:
            Out_TRNOutput.TRNHorUncertainty = hUncertainty * 6378000 * 25;
            Out_TRNOutput.TRNVerticalUncertainty = vUncertainty * 25;
            Out_TRNDatapump.xu = xu;
            Out_TRNDatapump.residual = residual;
            Out_Pmatrix = Pmatrix;
            %Out_TRNOutput.TRN_valid = TRN_valid;
            settings: executionOrder=3
        (default) -> AcquisitionCSU
        TrackingCSU -> AcquisitionCSU : [In_TRNOutput.NavigationMode == true]
        AcquisitionCSU -> TrackingCSU : [In_TRNOutput.NavigationMode == false]
      state Of_fTerrain_Map
      (default) -> On_Terrain_Map
      On_Terrain_Map -> Of_fTerrain_Map : [Out_TRNOutput.AircraftOffTerrainMap == true]
      Of_fTerrain_Map -> On_Terrain_Map : [Out_TRNOutput.AircraftOffTerrainMap == false]
  state Flight_Idle
    en, du:
    Out_TRNOutput.AircraftOffTerrainMap = CheckOffTerrainMap(In_TRNInput.Latitude_INS, In_TRNInput.Longitude_INS);
    Out_TRNOutput.TRN_valid = true;
    Out_TRNOutput.TRNEstOfINSLatitudeErr = 0.0;
    Out_TRNOutput.TRNEstOfINSLongitudeErr = 0.0;
    Out_TRNOutput.TRNEstOfINSAltitudeErr = 0.0;
    Out_TRNOutput.NavigationMode = false;
    Out_TRNOutput.AircraftPositionCorrectionValid = false;
  state [xu,Out_Pmatrix,residual,latINSErrTRN,lonINSErrTRN,altINSErrTRN,hUncertainty,vUncertainty,TimeTag_Prev,Result_Prev] = TrackingCSU(In_TRNInput,In_Pmatrix,Qmatrix,Rmatrix,In_TRNDatapump) [function]
  state [MAD,profileCnt,posUpdate,residual] = AcquisitionCSU(In_TRNInput,In_TRNDatapump) [function]
  (default) -> Operation_In_Flight
  Operation_In_Flight -> Flight_Idle : [In_TRNInput.WeightOnWheels == 1]
  Flight_Idle -> Operation_In_Flight : [In_TRNInput.WeightOnWheels == 0]
  data: In_TRNInput function_input Bus: TRNInput size=1 =0; In_Pmatrix function_input double size=[15 15]; Qmatrix function_input double size=[6 6]; Rmatrix function_input double size=1; xu function_output; Out_Pmatrix function_output; residual function_output; latINSErrTRN function_output; lonINSErrTRN function_output; altINSErrTRN function_output; hUncertainty function_output; vUncertainty function_output; In_TRNDatapump function_input Bus: TRNDatapump size=1; TimeTag_Prev function_output; Result_Prev function_output; In_TRNInput function_input Bus: TRNInput size=1 =0; In_TRNDatapump function_input Bus: TRNDatapump size=1 =0; MAD function_output; profileCnt function_output; posUpdate function_output; residual function_output; hUncertaintyTRN function_input; INSDataNotValid function_input; valid function_output; navigationMode function_output; Pmat function_output double size=[15 15]; lat function_input; lon function_input; AircraftOffTerrainMap function_output; In_TRNInput input Bus: TRNInput; In_TRNOutput input Bus: TRNOutput; In_TRNDatapump input Bus: TRNDatapump; In_Pmatrix input double size=[15 15]; Out_TRNOutput output Bus: TRNOutput; Out_TRNDatapump output Bus: TRNDatapump; Qmatrix input double size=[6 6]; Rmatrix input double size=1; vUncertainty local double; lonINSErrTRN local double; latINSErrTRN local double; hUncertainty local double; altINSErrTRN local double; posUpdate local double; continuousValid local boolean; residual local double; xu local double size=15; Pmatrix local double size=[15 15]; Out_Pmatrix output double size=[15 15]
  function [valid, navigationMode] = CheckValidity(hUncertaintyTRN, INSDataNotValid):
    | % function [valid, navigationMode] = CheckValidity(hUncertaintyTRN, vUncertaintyTRN, residualTRN)
    | 
    | % persistent invalidCnt
    | % if(isempty(invalidCnt))
    | %     invalidCnt = 0;
    | % end
    | % 
    | % weightedResidual = abs(residualTRN)/vUncertaintyTRN;
    | % 
    | % if(vUncertainty > 1 && weightedResidual > 35)
    | %     valid = false;
    | %     invalidCnt = invalidCnt + 1;
    | % else
    | %     valid = true;
    | %     invalidCnt = 0;
    | % end
    | % 
    | % if (invalidCnt >= 50)
    | %     navigationMode = true;
    | % else
    | %     navigationMode = false;
    | % end
    | % 
    | % end
    | 
    | function [valid, navigationMode] = CheckValidity(hUncertaintyTRN, INSDataNotValid)
    | 
    | persistent invalidCnt
    | if(isempty(invalidCnt))
    |     invalidCnt = 0;
    | end
    | 
    | if(hUncertaintyTRN > (256 * 6378000 * 25)) || INSDataNotValid == 1
    | % if(hUncertaintyTRN > (256))
    |     valid = false;
    |     invalidCnt = invalidCnt + 1;
    | else
    |     valid = true;
    |     invalidCnt = 0;
    | end
    | 
    | if (invalidCnt >= 50) || INSDataNotValid == 1
    |     navigationMode = true;        % Acq CSU
    | else
    |     navigationMode = false;       % Track CSU
    | end
    | 
    | end
  function Pmat = InitPmatrix:
    | function Pmat = InitPmatrix()
    | 
    | R0      = 6378000;
    | 
    | attBias = [0 0 0];
    | velBias = [0 0 0];
    | posBias = [10 10 13.3] .* [1/R0 1/R0 1];
    | gyroBias = [0.4848e-6 0.4848e-6 0.4848e-6];
    | accBias = [2.9430e-4 2.9430e-4 2.9430e-4];
    | 
    | % Pmat = diag(0.*[attBias velBias posBias gyroBias accBias].^2);
    | Pmat = diag([attBias velBias posBias gyroBias accBias].^2);
    | 
    | end
  function AircraftOffTerrainMap = CheckOffTerrainMap(lat, lon):
    | function AircraftOffTerrainMap = CheckOffTerrainMap(lat, lon)
    | 
    | AircraftTerrainMap = 0;
    | AircraftTerrainMap = coder.ceval('IsScanBoundary', lat, lon);     % InBoundary 1, NotBoundary 0
    | 
    | if(AircraftTerrainMap == 0)     % InBoundary 1, NotBoundary 0
    |     AircraftOffTerrainMap = true;
    | else
    |     AircraftOffTerrainMap = false;
    | end
    | 
    | end

== matlab function TRN_V3_CodeGen/TRN/TRNSchedulerDTNS1/AcquisitionCSU/AcquisitionCSU/CorrelationAnalysis function ==
  data: batchProfile input; posUpdate output; profileCnt input; MAD output; resolution input; gridSize input; residual output; batchProfile output; lonTemp output; latTemp output; hDEM output; sum output
function [posUpdate, MAD, residual, batchProfile, lonTemp,latTemp,hDEM, sum] = CorrelationAnalysis(batchProfile, profileCnt, resolution, gridSize)
r2d = 180/pi;

posUpdate   = zeros(2,1);
MAD         = single(0);
sum         = 0;
latTemp     = 0;
lonTemp     = 0;
hDEM        = 0;
bestIdx     = [-999 -999];

gridRes  = 0.1;
MADTemp = 9999*ones(1,8000);

for i = -gridSize : gridSize
    for j = -gridSize : gridSize
        
        latTemp = batchProfile(((profileCnt-1)*(3+(gridSize+gridSize+1)*(gridSize+gridSize+1))) + 2) + i*gridRes*resolution;
        lonTemp = batchProfile(((profileCnt-1)*(3+(gridSize+gridSize+1)*(gridSize+gridSize+1))) + 3) + j*gridRes*resolution;
        hDEM    = coder.ceval('GetElevation', latTemp*r2d, lonTemp*r2d);

        batchProfile(((profileCnt-1)*(3+(gridSize+gridSize+1)*(gridSize+gridSize+1))) + 3 + ((i + gridSize) * (gridSize+gridSize+1)) + (j + gridSize + 1)) = abs(batchProfile(((profileCnt-1)*(3+(gridSize+gridSize+1)*(gridSize+gridSize+1))) + 1) - hDEM );   
    end
end

for i = 1 : (gridSize+gridSize+1) * (gridSize+gridSize+1)
    sum = 0;
    for j = 1 : profileCnt
        sum = sum + batchProfile(((j-1)*(3+(gridSize+gridSize+1)*(gridSize+gridSize+1))) + (i+3));
    end
    
    MADTemp(1,i) = sum/single(profileCnt);
    
end

[minMAD, minIdx] = min(MADTemp);
MAD = single(minMAD);
bestIdx(1) = floor(minIdx/(gridSize+gridSize+1));
bestIdx(2) = minIdx - (bestIdx(1) * (gridSize+gridSize+1));

if bestIdx(2) == 0
    bestIdx(1) = bestIdx(1) - 1;
    bestIdx(2) = (gridSize+gridSize);
end
%
bestIdx(1) = bestIdx(1) - gridSize;
bestIdx(2) = bestIdx(2) - gridSize - 1;
posUpdate(1) = bestIdx(1)*gridRes*resolution;
posUpdate(2) = bestIdx(2)*gridRes*resolution;

residual = double(MAD);

end

== matlab function TRN_V3_CodeGen/TRN/TRNSchedulerDTNS1/TrackingCSU/TrackingCSU1/EKFupdate/MATLAB Function ==
  data: u input; y1 output; y2 output; y3 output
function [y1,y2,y3] = fcn(u)
    y = (u);
    yy = [y(7), y(8), y(9)];
    utm_lat2m_deg = 110961.7060516;   
    utm_lon2m_deg = 89476.51124;

    y1 = rad2deg(yy(1))*utm_lat2m_deg;
    y2 = rad2deg(yy(2))*utm_lon2m_deg;
    y3 = yy(3);

end

== matlab function TRN_V3_CodeGen/TRN/TRNSchedulerDTNS1/AcquisitionCSU/AcquisitionCSU/StoreProfile function ==
  data: batchProfile input; batchProfile output; profileCnt input; latINS input; lonINS input; altINS input; RALT input; profileCnt output; gridSize output; latGPS input; lonGPS input; altGPS input; flagGPS input; flagINS input
function [batchProfile, profileCnt, gridSize] = StoreProfile(batchProfile, profileCnt, latINS, lonINS, altINS, RALT, latGPS, lonGPS, altGPS, flagGPS, flagINS)

gridSize = 20;

if(profileCnt >= 20)
      
    profileCnt = uint32(19);
    
    for i = 0:profileCnt-1
   
        for j = 1 : (3 + (gridSize + gridSize + 1) * (gridSize + gridSize + 1))
            batchProfile(i * (3 + (gridSize + gridSize + 1) * (gridSize + gridSize + 1)) + j) = batchProfile((i+1) * (3 + (gridSize + gridSize + 1) * (gridSize + gridSize + 1)) + j);
        end
    end
            
end

if flagGPS == 1
    batchProfile((profileCnt*(3+((gridSize + gridSize + 1) * (gridSize + gridSize + 1)))) + 1) = altINS - RALT;
    batchProfile((profileCnt*(3+((gridSize + gridSize + 1) * (gridSize + gridSize + 1)))) + 2) = latINS;
    batchProfile((profileCnt*(3+((gridSize + gridSize + 1) * (gridSize + gridSize + 1)))) + 3) = lonINS;
elseif flagGPS == 0
    batchProfile((profileCnt*(3+((gridSize + gridSize + 1) * (gridSize + gridSize + 1)))) + 1) = altGPS - RALT;
    batchProfile((profileCnt*(3+((gridSize + gridSize + 1) * (gridSize + gridSize + 1)))) + 2) = latGPS;
    batchProfile((profileCnt*(3+((gridSize + gridSize + 1) * (gridSize + gridSize + 1)))) + 3) = lonGPS;
end

if flagINS == 0
    profileCnt = profileCnt + 1;
elseif flagINS == 1
    profileCnt = uint32(0);
end

end

== matlab function TRN_V3_CodeGen/TRN/TRNSchedulerDTNS1/TrackingCSU/TrackingCSU1/Earth_radius ==
  data: M output; N output; in_psi input
function [M, N] = Earth_radius(in_psi)

    a   = 6378137;          % Earth's equatorial radius
    b   = 6356752.314245;   % Earth's polar radius
    psi = in_psi;           % psi(latitude_GPS)
    M   = ((a*b)^2) / ( ( (a*cos(psi))^2 + (b*sin(psi))^2 )^(3/2) );    % radius  of  curvature  in  meridian
    N   = (a^2) / ( ( (a*cos(psi))^2 + (b*sin(psi))^2 )^(1/2) );        % radius  of  curvature  in  prime  vertical

end

== matlab function TRN_V3_CodeGen/TRN/TRNSchedulerDTNS1/TrackingCSU/TrackingCSU1/INS_Update_1553falt ==
  data: latINS input; latINS output; lonINS input; altINS input; velN input; velE input; velD input; TimeTag input; lonINS output; altINS output; dt input
function [latINS, lonINS, altINS] = fcn(latINS, lonINS, altINS, velN, velE, velD, TimeTag, dt)

R0 = 6378000;

if TimeTag(5) == 1
    latINS = latINS + (velN * dt) * 1/(R0+altINS);
    lonINS = lonINS + (velE * dt) * 1/(R0+altINS);
    altINS = altINS + (velD * dt) * 1/(R0+altINS);
end

== matlab function TRN_V3_CodeGen/TRN/RALTValidCheck/MATLAB Function6 ==
  data: residual input; sigma_3 input; RALT_valid output; count output; count input
function [RALT_valid, count] = RALTValidCheck(residual, sigma_3, count)

if abs(residual) >= sigma_3
    count = count + 1;
else
    count = 0;
end

if count > 7
    RALT_valid = boolean(false);
else
    RALT_valid = boolean(true);
end

== matlab function TRN_V3_CodeGen/TRN/INS//GPSFilter/MATLAB Function ==
  data: u input; yy output
function yy = fcn(u)
    y = diag(u);
    yy = [y(1), y(2), y(3)./(6378000)];

    yy = yy.*(6378000*25);

end

== matlab function TRN_V3_CodeGen/TRN/Multiple Model Adaptive Estimation ==
  data: WoW input; GPSDataNotValid input; TRN_INSEstErr input; out_Corr_Lat output; TRN_Pmat_Lat input; TRN_Pmat_Lon input; TRN_Pmat_Alt input; LCI_INSEstErr input; LCI_Pmat_Lat input; LCI_Pmat_Lon input; LCI_Pmat_Alt input; out_Corr_Lon output; out_Corr_Alt output; Weight output
function [out_Corr_Lat,out_Corr_Lon,out_Corr_Alt,Weight] = MMAE(WoW, GPSDataNotValid,TRN_INSEstErr,TRN_Pmat_Lat,TRN_Pmat_Lon,TRN_Pmat_Alt,LCI_INSEstErr,LCI_Pmat_Lat,LCI_Pmat_Lon,LCI_Pmat_Alt)

Weight_Lat   = TRN_Pmat_Lat/(LCI_Pmat_Lat+TRN_Pmat_Lat);
Weight_Lon   = TRN_Pmat_Lon/(LCI_Pmat_Lon+TRN_Pmat_Lon);
Weight_Alt   = TRN_Pmat_Alt/(LCI_Pmat_Alt+TRN_Pmat_Alt);

if GPSDataNotValid == 0 && WoW == 0     % TRN+INS/GPS
    out_Corr_Lat = (1-Weight_Lat)*TRN_INSEstErr(1) + Weight_Lat*LCI_INSEstErr(1);
    out_Corr_Lon = (1-Weight_Lon)*TRN_INSEstErr(2) + Weight_Lon*LCI_INSEstErr(2);
    out_Corr_Alt = (1-Weight_Alt)*TRN_INSEstErr(3) + Weight_Alt*LCI_INSEstErr(3);
else                                    % TRN
    out_Corr_Lat = TRN_INSEstErr(1);
    out_Corr_Lon = TRN_INSEstErr(2);
    out_Corr_Alt = TRN_INSEstErr(3);
end

Weight = [Weight_Lat Weight_Lon Weight_Alt];

== matlab function TRN_V3_CodeGen/TRN/TRNSchedulerDTNS1/TrackingCSU/TrackingCSU1/MATLAB Function1 ==
  data: Lat_GPS input; Lon_GPS input; Alt_GPS input; Lat output; Lat_INS input; Lon_INS input; Alt_INS input; GPSvalid input; Lon output; Alt output
function [Lat,Lon,Alt] = fcn(Lat_GPS,Lon_GPS,Alt_GPS,Lat_INS,Lon_INS,Alt_INS,GPSvalid)

if GPSvalid == 0
    Lat = Lat_GPS;
    Lon = Lon_GPS;
    Alt = Alt_GPS;
else
    Lat = Lat_INS;
    Lon = Lon_INS;
    Alt = Alt_INS;
end

== matlab function TRN_V3_CodeGen/TRN/TRNSchedulerDTNS1/TrackingCSU/TrackingCSU1/MATLAB Function2 ==
  data: TimeTag_Prev input; TimeTag_Prev output; GPSTimeTag input; INSTimeTag input; RALTTimeTag input
function TimeTag_Prev   = fcn(TimeTag_Prev,GPSTimeTag,INSTimeTag,RALTTimeTag)


TimeTag_Prev(4) = 0;
TimeTag_Prev(5) = 0;
TimeTag_Prev(6) = 0;

if TimeTag_Prev(1) == GPSTimeTag
    TimeTag_Prev(4) = 1;
end

if TimeTag_Prev(2) == INSTimeTag
    TimeTag_Prev(5) = 1;
end

if TimeTag_Prev(3) == RALTTimeTag
    TimeTag_Prev(6) = 1;
end

TimeTag_Prev(1) = GPSTimeTag;
TimeTag_Prev(2) = INSTimeTag;
TimeTag_Prev(3) = RALTTimeTag;

== matlab function TRN_V3_CodeGen/TRN/INS//GPSFilter/Fupdate Function ==
  data: velN input; Fmatrix output; velE input; velD input; lat input; alt input; accN input; accE input; accD input; OM input; M input; N input
% ---------------------------------------------------------------------- %
%                   F matrix update function
%
%   INPUT:
%       velN: North Velocity                                [m/s]
%       velE: East Velocity                                 [m/s]
%       velD: Down Velocity                                 [m/s]
%       lat: Latitude                                       [rad]
%       alt: Altitude                                       [m]
%       accN: North acceleration                            [m/ss]
%       accE: East acceleration                             [m/ss]
%       accD: Down acceleration                             [m/ss]
%       OM: Magnitude of the rotation rate of the Earth     [rad/s]
%       DCMbn: Rotational matrix(body frame to navigation frame)
%       M: radius  of  curvature  in  meridian
%       N: radius  of  curvature  in  prime  vertical      
%
%   OUTPUT:
%       Fmatrix: System matrix of Kalman Filter
%
% ---------------------------------------------------------------------- %
function Fmatrix = Fupdate(velN, velE, velD, lat, alt, accN, accE, accD, OM, M, N)

    e11 = 0;
    e12 = -((OM * sin(lat)) + (velE/(N+alt) * tan(lat)));
    e13 = velN/(M+alt);
    e21 = ((OM * sin(lat)) + (velE/(N+alt) * tan(lat)));
    e22 = 0;
    e23 = ((OM * cos(lat)) + (velE/(N+alt)));
    e31 = -velN/(M+alt);
    e32 = -(OM * cos(lat)) - (velE/(N+alt));
    e33 = 0;
    Fee = [e11 e12 e13; e21 e22 e23; e31 e32 e33;];
    
    e11 = 0;
    e12 = 1/((N+alt));
    e13 = 0;
    e21 = -1/((M+alt));
    e22 = 0 ;
    e23 = 0 ;
    e31 = 0 ;
    e32 = -tan(lat)/(N+alt) ;
    e33 = 0 ;
    Fev = [e11 e12 e13; e21 e22 e23; e31 e32 e33;];
    
    e11 = -OM * sin(lat);
    e12 = 0;
    e13 = -velE/(((N+alt))^2);
    e21 = 0 ;
    e22 = 0 ;
    e23 = velN/(((M+alt))^2);
    e31 =  -(OM*cos(lat)) - (velE/(((N+alt))*(cos(lat))^2));
    e32 = 0 ;
    e33 = (velE * tan(lat)) / ((N+alt)^2) ;
    Fer = [e11 e12 e13; e21 e22 e23; e31 e32 e33;];
    
    e11 = 0 ;
    e12 = -accD ;
    e13 = accE ;
    e21 = accD ;
    e22 = 0 ;
    e23 = -accN ;
    e31 = -accE ;
    e32 = accN ;
    e33 = 0 ;
    Fve = [e11 e12 e13; e21 e22 e23; e31 e32 e33;];
    
    e11 = velD/((M+alt));
    e12 = -2*((OM * sin(lat)) + ((velE/((N+alt))) * tan (lat))) ;
    e13 = velN/(M+alt) ;
    e21 = (2*OM * sin(lat)) + ( (velE/((N+alt))) * tan(lat) );
    e22 = (1/((N+alt))) * ((velN * tan(lat)) + velD) ;
    e23 = 2*OM * cos(lat) + (velE/((N+alt)));
    e31 = (-2*velN)/((M+alt));
    e32 = -2*(OM * cos(lat) +  (velE/((N+alt)))) ;
    e33 = 0;
    Fvv = [e11 e12 e13; e21 e22 e23; e31 e32 e33;];
    
    e11 = -velE*( (2*OM * cos(lat)) + (velE/(((N+alt))*(cos(lat))^2)));
    e12 = 0 ;
    e13 = (((velE^2)*tan(lat))/((N+alt)^2)) - ((velN*velD)/((M+alt)^2)) ;
    e21 = 2*OM *((velN*cos(lat)) - (velD*sin(lat))) + ((velN*velE) / (((N+alt))*(cos(lat))^2)) ;
    e22 = 0 ;
    e23 = ((-velE*velD)/((N+alt)^2))-((velN*velE*tan(lat))/((N+alt)^2));
    e31 = 2 * OM * velE * sin(lat);
    e32 = 0;
    e33 =  (((velE^2)/((N+alt)^2)) + ((velN^2)/((M+alt)^2)));
    Fvr = [e11 e12 e13; e21 e22 e23; e31 e32 e33;];
    
    Fre = zeros(3);
    
    e11 = 1/((M+alt));
    e12 = 0;
    e13 = 0;
    e21 = 0;
    e22 = 1/(((N+alt))*cos(lat));
    e23 = 0;
    e31 = 0;
    e32 = 0;
    e33 = -1;
    Frv = [e11 e12 e13; e21 e22 e23; e31 e32 e33;];
    
    e11 = 0;
    e12 = 0;
    e13 = -velN/(((M+alt))^2);
    e21 = (velE*tan(lat))/(((N+alt))*cos(lat));
    e22 = 0;
    e23 = -velE/((((N+alt))^2)*cos(lat));
    e31 = 0;
    e32 = 0;
    e33 = 0;
    Frr = [e11 e12 e13; e21 e22 e23; e31 e32 e33;];
              
    Fmatrix =  [Frr    Frv    Fre      ;
                Fvr    Fvv    Fve      ;
                Fer    Fev    Fee      ];
        
end

== matlab function TRN_V3_CodeGen/TRN/INS//GPSFilter/Gupdate Function ==
  data: DCMbn input; Gmatrix output
% ---------------------------------------------------------------------- %
%                   G matrix update function
%
%   INPUT:
%       DCMbn: Rotational matrix(body frame to navigation frame)
%
%   OUTPUT:
%       Gmatrix: Input matrix of Kalman Filter
%
% ---------------------------------------------------------------------- %
function Gmatrix = Gupdate(DCMbn)

Z  = zeros(3);

Gmatrix =  [    Z       Z;
              DCMbn     Z;
                Z    -DCMbn;];

end
